simulink model "rosTest"  (R2021a)
settings: Solver=VariableStepAuto  StartTime=0.0  StopTime=inf  RelTol=1e-3
values from neighbouring files (symbols this model uses):
  s = 1/(2*r)    [Weg0.m]
undefined symbols (not defined in the file or in its folder): X, Y, Z
libraries: sm_lib x8, TripedLibrary x8, spsFirstOrderFilterLib x4, nesl_utility x4
settings Model: Creator=maxde  LastModifiedBy=maxde

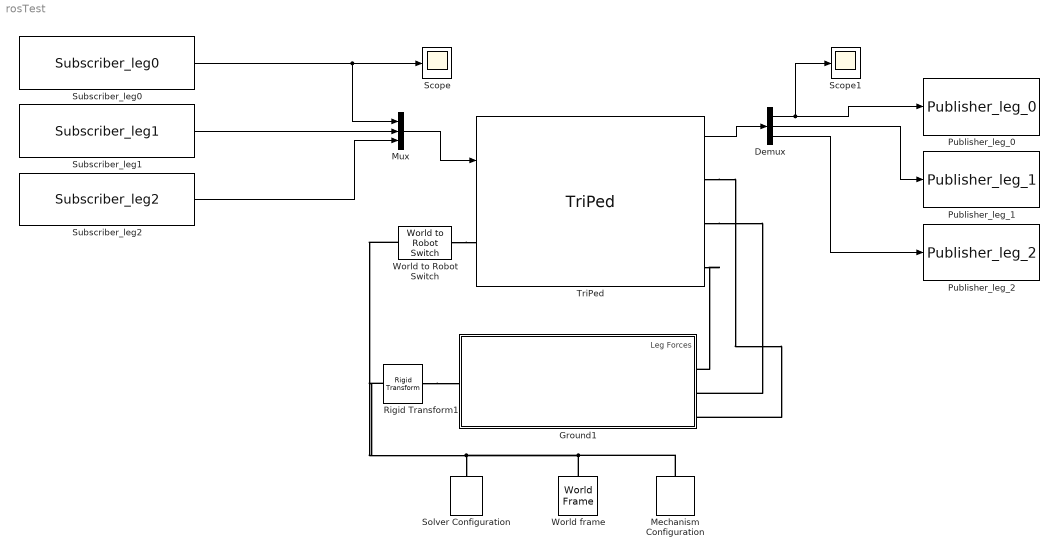
== system rosTest ==
  Demux : Demux  Outputs=3
  Ground1 : Subsystem
  Mechanism Configuration : sm_lib/Utilities/Mechanism Configuration  UniformGravity=Constant  GravityVector=[0 0 -9.80665]  GravityVectorUnits=m/s^2  GravityUnits=m/s^2  LinearizationDelta=0.001  JointModeTransitionNonlinearIterations=2
  Mux : Mux  Inputs=3
  Publisher_leg_0 : TripedLibrary/Full Model/ROS/Publishers/Publisher_leg_0  SystemSampleTime=-1  VariantActivationTime=update diagram  Latency=0  AutoFrameSizeCalculation=off
      settings: SourceProductName=TriPed Library
  Publisher_leg_1 : TripedLibrary/Full Model/ROS/Publishers/Publisher_leg_1  SystemSampleTime=-1  VariantActivationTime=update diagram  Latency=0  AutoFrameSizeCalculation=off
      settings: SourceProductName=TriPed Library
  Publisher_leg_2 : TripedLibrary/Full Model/ROS/Publishers/Publisher_leg_2  SystemSampleTime=-1  VariantActivationTime=update diagram  Latency=0  AutoFrameSizeCalculation=off
      settings: SourceProductName=TriPed Library
  Rigid Transform1 : sm_lib/Frames and Transforms/Rigid Transform  TranslationMethod=Cartesian  TranslationStandardOffset=-0.7  TranslationLengthUnit=m  TranslationStandardAxis=+Z  TranslationCartesianOffset="[1.5  0 -0.7]"  TranslationROffset=0  TranslationROffsetUnits=m  TranslationZOffset=0  TranslationZOffsetUnits=m  TranslationThetaOffset=0  TranslationThetaOffsetUnits=deg  RotationMethod=None  RotationAngleUnits=deg  RotationStandardAxis=+Z  RotationAngle=0.0  RotationArbitraryAxis=[0 0 1]  FollAlignAxisA=+X  BaseAlignAxisA=+Y  FollAlignAxisB=+Y  BaseAlignAxisB=+Z  RotationSequenceAxes=FollowerAxes  RotationSequence=XYX  RotationSequenceAngles=[0 0 0]  RotationSequenceAnglesUnits=deg  RotationMatrix=[1 0 0; 0 1 0; 0 0 1]
  Scope : Scope
  Scope1 : Scope
  Solver Configuration : nesl_utility/Solver Configuration  PhysicalDomain=network_engine_domain  SubClassName=solver  LeftPortType=input  RightPortType=generic  Tones=[]  Harmonics=[]  SimulateNoise=off  Profile=off  UseLocalSampling=off  EnableSwitchedLinearOptims=on  FrequencyDomain=off  UseCCode=off  RelTol=0.001  AbsTol=1e-06  MinStep=1e-09  ToWorkspace=off  RevertToSquareIcSolve=off  NumHomotopyIterations=100  PhasorMode=off  PhasorModeNumHarmonics=1  DoDC=off  ResidualTolerance=1e-06  UseLocalSolver=off  LocalSolverChoice=NE_BACKWARD_EULER_ADVANCER  LocalSolverSampleTime=0.001  DoFixedCost=off  MaxNonlinIter=3  MaxModeIter=2  ComputeImpulses=off  ImpulseIterations=2  LinearAlgebra=Sparse  EquationFormulation=NE_TIME_EF  DelaysMemoryBudget=1024  AutomaticFiltering=on  FilteringTimeConstant=0.001  PartitionStorageMethod=AS_NEEDED  PartitionMemoryBudget=1024  PartitionMethod=FAST
  Subscriber_leg0 : TripedLibrary/Full Model/ROS/Subscribers/Subscriber_leg0  SystemSampleTime=-1  VariantActivationTime=update diagram  Latency=0  AutoFrameSizeCalculation=off
      settings: SourceProductName=TriPed Library
  Subscriber_leg1 : TripedLibrary/Full Model/ROS/Subscribers/Subscriber_leg1  SystemSampleTime=-1  VariantActivationTime=update diagram  Latency=0  AutoFrameSizeCalculation=off
      settings: SourceProductName=TriPed Library
  Subscriber_leg2 : TripedLibrary/Full Model/ROS/Subscribers/Subscriber_leg2  SystemSampleTime=-1  VariantActivationTime=update diagram  Latency=0  AutoFrameSizeCalculation=off
      settings: SourceProductName=TriPed Library
  TriPed : TripedLibrary/Full Model/TriPed  SystemSampleTime=-1  VariantActivationTime=update diagram  Latency=0  AutoFrameSizeCalculation=off
      settings: SourceProductName=TriPed Library
  World frame : sm_lib/Frames and Transforms/World Frame
  World to Robot Switch : TripedLibrary/Environment/World to Robot Switch  SystemSampleTime=-1  LabelModeActiveChoice=(default)  VariantActivationTime=update diagram  Latency=0  AutoFrameSizeCalculation=off
      settings: SourceProductName=TriPed Library
  wires:
  Demux/1 -> Scope1/1, Publisher_leg_0/1
  Demux/2 -> Publisher_leg_1/1
  Demux/3 -> Publisher_leg_2/1
  TriPed/1 -> Demux/1
  Subscriber_leg0/1 -> Mux/1, Scope/1
  Mux/1 -> TriPed/1
  Subscriber_leg1/1 -> Mux/2
  Subscriber_leg2/1 -> Mux/3
  connections:
  Mechanism Configuration/RConn1 -- World frame/RConn1 -- World to Robot Switch/LConn1 -- Rigid Transform1/LConn1 -- Solver Configuration/RConn1
  TriPed/RConn3 -- Ground1/RConn1
  Rigid Transform1/RConn1 -- Ground1/LConn1
  TriPed/RConn2 -- Ground1/RConn2
  TriPed/RConn1 -- Ground1/RConn3
  World to Robot Switch/RConn1 -- TriPed/LConn1

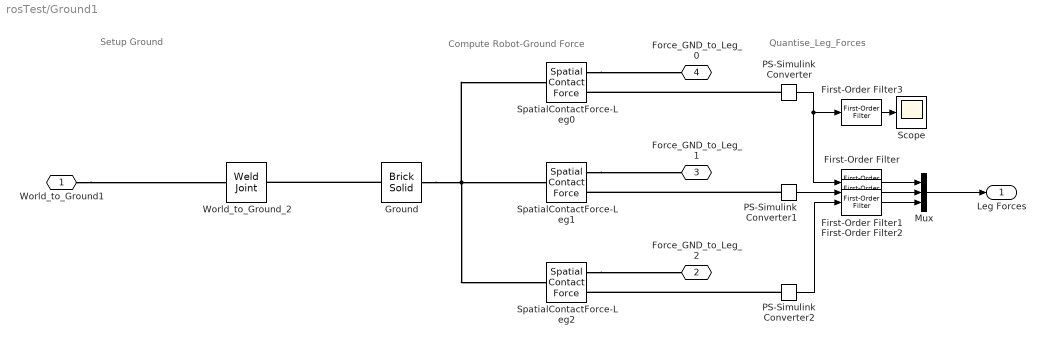
== system rosTest/Ground1 ==
  note: Setup Ground
  note: Compute Robot-Ground Force
  note: Quantise_Leg_Forces
  First-Order Filter : spsFirstOrderFilterLib/First-Order Filter  FilterType=Lowpass  Tc=1/30  Ts=0  Initialize=on  Vac_Init=[0, 0, 60]  Vdc_Init=0  PlotResponse=off  FreqRange="[0,  200,  1]"
  First-Order Filter1 : spsFirstOrderFilterLib/First-Order Filter  FilterType=Lowpass  Tc=1/30  Ts=0  Initialize=on  Vac_Init=[0, 0, 60]  Vdc_Init=0  PlotResponse=off  FreqRange="[0,  200,  1]"
  First-Order Filter2 : spsFirstOrderFilterLib/First-Order Filter  FilterType=Lowpass  Tc=1/30  Ts=0  Initialize=on  Vac_Init=[0, 0, 60]  Vdc_Init=0  PlotResponse=off  FreqRange="[0,  200,  1]"
  First-Order Filter3 : spsFirstOrderFilterLib/First-Order Filter  FilterType=Lowpass  Tc=1/5  Ts=0  Initialize=on  Vac_Init=[0, 0, 60]  Vdc_Init=0  PlotResponse=off  FreqRange="[0,  200,  1]"
  Ground : sm_lib/Body Elements/Brick Solid  GraphicAmbientColor=[0.15 0.15 0.15 1.0]  BasedOnType=Density  BrickDimensions=[5 5 0.1]  BrickDimensionUnits=m  CenterOfMass=[0 0 0]  CenterOfMassUnits=m  GraphicDiffuseColor=[0.4 0.4 0.4]  Density=1000  DensityUnits=kg/m^3  DoExposeReferenceFrame=on  GraphicEmissiveColor=[0.0 0.0 0.0 1.0]  ExportEntireGeometry=on  SerializedFrames=<Frames/>  MarkerShape=Sphere  MarkerSize=10  GraphicType=FromGeometry  InertiaType=CalculateFromGeometry  Mass=1  MassUnits=kg  MomentsOfInertia=[1 1 1]  MomentsOfInertiaUnits=kg*m^2  GraphicOpacity=0.8  ProductsOfInertia=[0 0 0]  ProductsOfInertiaUnits=kg*m^2  GraphicShininess=75  GraphicSpecularColor=[0.5 0.5 0.5 1.0]  GraphicVisPropType=SimpleVisualProperties
  Mux : Mux  Inputs=3
  PS-Simulink Converter : nesl_utility/PS-Simulink Converter  PhysicalDomain=network_engine_domain  SubClassName=ps_output  LeftPortType=input  RightPortType=output  PseudoPeriodic=off  Frequencies=[]  Unit=inherit  AffineConversion=off
  PS-Simulink Converter1 : nesl_utility/PS-Simulink Converter  PhysicalDomain=network_engine_domain  SubClassName=ps_output  LeftPortType=input  RightPortType=output  PseudoPeriodic=off  Frequencies=[]  Unit=inherit  AffineConversion=off
  PS-Simulink Converter2 : nesl_utility/PS-Simulink Converter  PhysicalDomain=network_engine_domain  SubClassName=ps_output  LeftPortType=input  RightPortType=output  PseudoPeriodic=off  Frequencies=[]  Unit=inherit  AffineConversion=off
  Scope : Scope
  SpatialContactForce-Leg0 : sm_lib/Forces and Torques/Spatial Contact Force  CoefficientOfDynamicFriction=0.6  CoefficientOfStaticFriction=1  SenseContactBaseRotation=off  SenseContactBaseTranslation=off  NormalDamping=10^3  NormalDampingUnits=N/(m/s)  SenseContactFollowerRotation=off  SenseContactFollowerTranslation=off  SenseContactSignal=off  NormalStiffness=30000  NormalStiffnessUnits=N/m  FrictionalCriticalVelocity=1e-2  FrictionalCriticalVelocityUnits=m/s  ZeroCrossDetectContactStartAndEnd=on  FrictionType=SmoothStickSlip  SenseFrictionalForceMagnitude=off  SenseNormalForceMagnitude=on  NormalForceType=SmoothSpringDamper  SenseNormalVelocity=off  SenseSeparationDistance=off  SenseTangentialVelocity=off  SenseTangentialVelocityMagnitude=off  NormalTransitionRegionWidth=1e-3  NormalTransitionRegionWidthUnits=m
  SpatialContactForce-Leg1 : sm_lib/Forces and Torques/Spatial Contact Force  CoefficientOfDynamicFriction=0.6  CoefficientOfStaticFriction=1  SenseContactBaseRotation=off  SenseContactBaseTranslation=off  NormalDamping=10^3  NormalDampingUnits=N/(m/s)  SenseContactFollowerRotation=off  SenseContactFollowerTranslation=off  SenseContactSignal=off  NormalStiffness=30000  NormalStiffnessUnits=N/m  FrictionalCriticalVelocity=1e-2  FrictionalCriticalVelocityUnits=m/s  ZeroCrossDetectContactStartAndEnd=on  FrictionType=SmoothStickSlip  SenseFrictionalForceMagnitude=off  SenseNormalForceMagnitude=on  NormalForceType=SmoothSpringDamper  SenseNormalVelocity=off  SenseSeparationDistance=off  SenseTangentialVelocity=off  SenseTangentialVelocityMagnitude=off  NormalTransitionRegionWidth=1e-3  NormalTransitionRegionWidthUnits=m
  SpatialContactForce-Leg2 : sm_lib/Forces and Torques/Spatial Contact Force  CoefficientOfDynamicFriction=0.6  CoefficientOfStaticFriction=1  SenseContactBaseRotation=off  SenseContactBaseTranslation=off  NormalDamping=10^3  NormalDampingUnits=N/(m/s)  SenseContactFollowerRotation=off  SenseContactFollowerTranslation=off  SenseContactSignal=off  NormalStiffness=30000  NormalStiffnessUnits=N/m  FrictionalCriticalVelocity=1e-2  FrictionalCriticalVelocityUnits=m/s  ZeroCrossDetectContactStartAndEnd=on  FrictionType=SmoothStickSlip  SenseFrictionalForceMagnitude=off  SenseNormalForceMagnitude=on  NormalForceType=SmoothSpringDamper  SenseNormalVelocity=off  SenseSeparationDistance=off  SenseTangentialVelocity=off  SenseTangentialVelocityMagnitude=off  NormalTransitionRegionWidth=1e-3  NormalTransitionRegionWidthUnits=m
  World_to_Ground_2 : sm_lib/Joints/Weld Joint  JointMode=Normal  SenseConstraintForce=off  SenseConstraintForceX=off  SenseConstraintForceY=off  SenseConstraintForceZ=off  SenseConstraintTorque=off  SenseConstraintTorqueX=off  SenseConstraintTorqueY=off  SenseConstraintTorqueZ=off  SenseTotalForce=off  SenseTotalForceX=off  SenseTotalForceY=off  SenseTotalForceZ=off  SenseTotalTorque=off  SenseTotalTorqueX=off  SenseTotalTorqueY=off  SenseTotalTorqueZ=off  CompositeWrenchDir=FollowerOnBase  CompositeWrenchFrame=BaseFrame
  World_to_Ground1 : PMIOPort  Side=Left
  Force_GND_to_Leg_2 : PMIOPort  Port=2  Side=Right
  Force_GND_to_Leg_1 : PMIOPort  Port=3  Side=Right
  Force_GND_to_Leg_0 : PMIOPort  Port=4  Side=Right
  Leg Forces : Outport
  wires:
  PS-Simulink Converter/1 -> First-Order Filter3/1, First-Order Filter/1
  PS-Simulink Converter1/1 -> First-Order Filter1/1
  PS-Simulink Converter2/1 -> First-Order Filter2/1
  Mux/1 -> Leg Forces/1
  First-Order Filter/1 -> Mux/1
  First-Order Filter1/1 -> Mux/2
  First-Order Filter2/1 -> Mux/3
  First-Order Filter3/1 -> Scope/1
  connections:
  Ground/RConn1 -- World_to_Ground_2/RConn1
  Ground/LConn1 -- SpatialContactForce-Leg0/LConn1 -- SpatialContactForce-Leg1/LConn1 -- SpatialContactForce-Leg2/LConn1
  SpatialContactForce-Leg1/RConn1 -- Force_GND_to_Leg_1/RConn1
  SpatialContactForce-Leg2/RConn1 -- Force_GND_to_Leg_2/RConn1
  SpatialContactForce-Leg0/RConn1 -- Force_GND_to_Leg_0/RConn1
  World_to_Ground1/RConn1 -- World_to_Ground_2/LConn1
  PS-Simulink Converter1/LConn1 -- SpatialContactForce-Leg1/RConn2
  PS-Simulink Converter2/LConn1 -- SpatialContactForce-Leg2/RConn2
  PS-Simulink Converter/LConn1 -- SpatialContactForce-Leg0/RConn2
